simulink model "FDIteamUAV"  (R2018a)
settings: Solver=FixedStepAuto  StartTime=0.0  StopTime=100  FixedStep=0.1  RelTol=1e-3
InitFcn:
  | clear
  | close all
  | parameterVehicleControl
  | fdi_mask_init
values from neighbouring files (symbols this model uses):
  a = x_waypoint(1)+10    [parameterVehicleControl.m]
  a2 = x_waypoint(1)    [parameterVehicleControl.m]
  a3 = x_waypoint(1)-10    [parameterVehicleControl.m]
  b = y_waypoint(1)    [parameterVehicleControl.m]
  b2 = y_waypoint(1)    [parameterVehicleControl.m]
  b3 = y_waypoint(1)    [parameterVehicleControl.m]
  fdi_alarm_thrsld = 9.2103    [fdi_mask_init.m]
  fdi_duration_1_airs = 55    [fdi_mask_init.m]
  fdi_duration_2_airs = 1000    [fdi_mask_init.m]
  fdi_duration_3_airs = 0    [fdi_mask_init.m]
  fdi_fixed_matix_1_airs = fdi_fault_value_1_airs    (= 3)    [fdi_mask_init.m]
  fdi_fixed_matix_2_airs = fdi_fault_value_2_airs    (= 3)    [fdi_mask_init.m]
  fdi_fixed_matix_3_airs = fdi_fault_value_3_airs    (= 0)    [fdi_mask_init.m]
  fdi_gain_matrix_1_airs = 1    [fdi_mask_init.m]
  fdi_gain_matrix_2_airs = 1    [fdi_mask_init.m]
  fdi_gain_matrix_3_airs = 1    [fdi_mask_init.m]
  fdi_muNmu_1_airs = fdi_mu_1_airs/norm(fdi_mu_1_airs)    [fdi_mask_init.m]
  fdi_muNmu_2_airs = fdi_mu_2_airs/norm(fdi_mu_2_airs)    [fdi_mask_init.m]
  fdi_muNmu_3_airs = fdi_mu_3_airs/norm(fdi_mu_3_airs)    [fdi_mask_init.m]
  fdi_noise_var_airs = Noise_airs    (= 0.2)    [fdi_mask_init.m]
  fdi_seed_airs = ceil(rand(1,fdi_number_of_sensors)*1000)    [fdi_mask_init.m]
  fdi_SmT_airs = (fdi_V * fdi_R_airs * fdi_V')^(-1/2)    [fdi_mask_init.m]
  fdi_start_time_1_airs = 45    [fdi_mask_init.m]
  fdi_start_time_2_airs = 500    [fdi_mask_init.m]
  fdi_start_time_3_airs = 0    [fdi_mask_init.m]
  fdi_V = (null([1 1 1]))'    [fdi_mask_init.m]
  rl = 1*rNominal    (= 0.052959)    [parameterVehicleControl.m]
  rr = 1*rNominal    (= 0.052959)    [parameterVehicleControl.m]
  Tau2 = 1    [parameterVehicleControl.m]
  thetaIC = 90*(pi/180)    (= 1.57079632679)    [parameterVehicleControl.m]
  thetaIC2 = 90*(pi/180)    (= 1.57079632679)    [parameterVehicleControl.m]
  thetaIC3 = 90*(pi/180)    (= 1.57079632679)    [parameterVehicleControl.m]
  Ts = Tsample    [fdi_mask_init.m]
  Tsample = 1/10    (= 0.1)    [parameterVehicleControl.m]
  Vmax = 5    [parameterVehicleControl.m]
  xIC = 150    [parameterVehicleControl.m]
  xIC2 = 25    [parameterVehicleControl.m]
  xIC3 = -100    [parameterVehicleControl.m]
  yIC = 0    [parameterVehicleControl.m]
  yIC2 = 0    [parameterVehicleControl.m]
  yIC3 = 0    [parameterVehicleControl.m]
libraries: simulink x6
settings Model: Creator=hsevil  LastModifiedBy=hsevil
settings SolverCC: AlgebraicLoopSolver=LineSearch

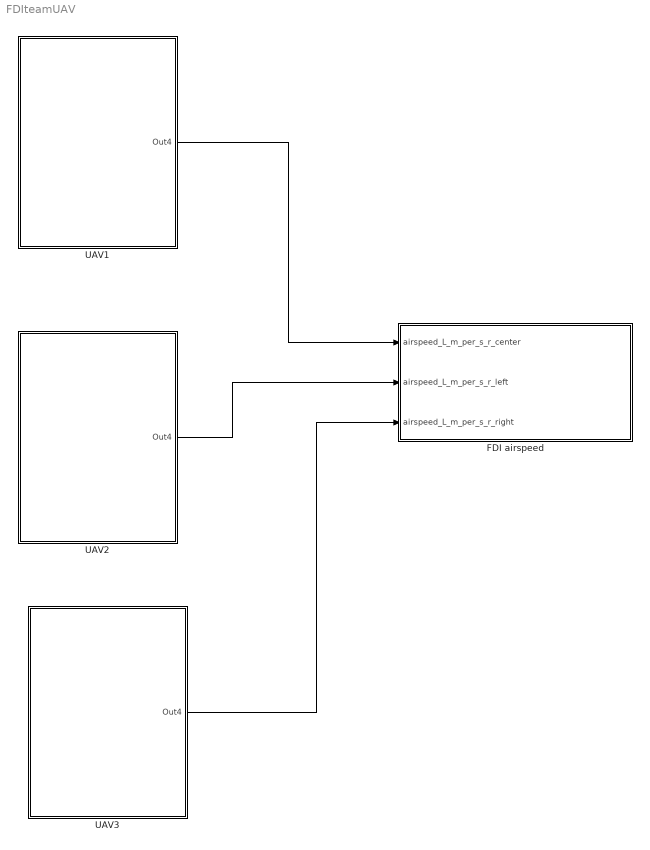
== system FDIteamUAV ==
  FDI airspeed : Subsystem
  UAV1 : Subsystem
  UAV2 : Subsystem
  UAV3 : Subsystem
  wires:
  UAV1/1(Out4) -> FDI airspeed/1(airspeed_L_m_per_s_r_center)
  UAV2/1(Out4) -> FDI airspeed/2(airspeed_L_m_per_s_r_left)
  UAV3/1(Out4) -> FDI airspeed/3(airspeed_L_m_per_s_r_right)

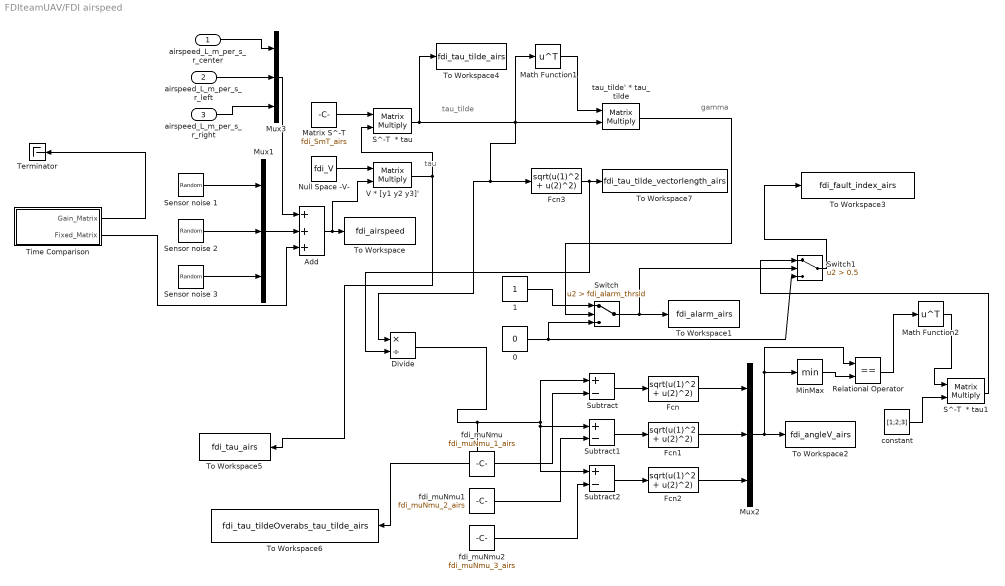
== system FDIteamUAV/FDI airspeed ==
  note: tau
  note: gamma
  note: tau_tilde
  airspeed_L_m_per_s_r_center : Inport
  airspeed_L_m_per_s_r_left : Inport  Port=2
  airspeed_L_m_per_s_r_right : Inport  Port=3
  0 : Constant  Value=0
  1 : Constant
  Add : Sum  Inputs=+++
  Divide : Product  Inputs=*/
  Fcn{,1..3} (4 alike) : Fcn  Expr=sqrt(u(1)^2 + u(2)^2)
  Math Function1 : Math  Operator=transpose  SaturateOnIntegerOverflow=on
  Math Function2 : Math  Operator=transpose  SaturateOnIntegerOverflow=on
  Matrix S^-T : Constant  Value=fdi_SmT_airs
  MinMax : MinMax
  Mux1 : Mux  Inputs=3
  Mux2 : Mux  Inputs=3
  Mux3 : Mux  Inputs=3
  Null Space -V- : Constant  Value=fdi_V
  Relational Operator : RelationalOperator  Operator===  OutDataTypeStr=boolean  RndMeth=Nearest
  S^-T  * tau : Product  Multiplication=Matrix(*)  RndMeth=Zero
  S^-T  * tau1 : Product  Multiplication=Matrix(*)  RndMeth=Zero
  Sensor noise 1 : RandomNumber  DisableCoverage=on  Variance=fdi_noise_var_airs  Seed=fdi_seed_airs(1)  SampleTime=Ts
  Sensor noise 2 : RandomNumber  DisableCoverage=on  Variance=fdi_noise_var_airs  Seed=fdi_seed_airs(2)  SampleTime=Ts
  Sensor noise 3 : RandomNumber  DisableCoverage=on  Variance=fdi_noise_var_airs  Seed=fdi_seed_airs(3)  SampleTime=Ts
  Subtract : Sum  Inputs=+-
  Subtract1 : Sum  Inputs=+-
  Subtract2 : Sum  Inputs=+-
  Switch : Switch  Criteria=u2 > Threshold  Threshold=fdi_alarm_thrsld
  Switch1 : Switch  Criteria=u2 > Threshold  Threshold=0.5
  Terminator : Terminator
  Time Comparison : Subsystem
  To Workspace : ToWorkspace  VariableName=fdi_airspeed  SampleTime=-1
  To Workspace1 : ToWorkspace  VariableName=fdi_alarm_airs  SampleTime=-1
  To Workspace2 : ToWorkspace  VariableName=fdi_angleV_airs  SampleTime=-1
  To Workspace3 : ToWorkspace  VariableName=fdi_fault_index_airs  SampleTime=-1
  To Workspace4 : ToWorkspace  VariableName=fdi_tau_tilde_airs  SampleTime=-1
  To Workspace5 : ToWorkspace  VariableName=fdi_tau_airs  SampleTime=-1
  To Workspace6 : ToWorkspace  VariableName=fdi_tau_tildeOverabs_tau_tilde_airs  SampleTime=-1
  To Workspace7 : ToWorkspace  VariableName=fdi_tau_tilde_vectorlength_airs  SampleTime=-1
  V * [y1 y2 y3]' : Product  Multiplication=Matrix(*)  RndMeth=Zero
  constant : Constant  Value=[1;2;3]
  fdi_muNmu : Constant  Value=fdi_muNmu_1_airs
  fdi_muNmu1 : Constant  Value=fdi_muNmu_2_airs
  fdi_muNmu2 : Constant  Value=fdi_muNmu_3_airs
  tau_tilde' * tau_tilde : Product  Multiplication=Matrix(*)  RndMeth=Zero
  wires:
  Sensor noise 1/1 -> Mux1/1
  Sensor noise 2/1 -> Mux1/2
  Sensor noise 3/1 -> Mux1/3
  Mux1/1 -> Add/2
  Mux3/1 -> Add/1
  Add/1 -> To Workspace/1, V * [y1 y2 y3]'/2
  Null Space -V-/1 -> V * [y1 y2 y3]'/1
  V * [y1 y2 y3]'/1 -> S^-T  * tau/2, To Workspace5/1
  Switch/1 -> To Workspace1/1, Switch1/2
  Math Function1/1 -> tau_tilde' * tau_tilde/1
  tau_tilde' * tau_tilde/1 -> Switch/2
  1/1 -> Switch/1
  0/1 -> Switch/3, Switch1/3
  S^-T  * tau/1 -> To Workspace4/1, Fcn3/1, Divide/1, tau_tilde' * tau_tilde/2, Math Function1/1
  Matrix S^-T/1 -> S^-T  * tau/1
  Subtract/1 -> Fcn/1
  Subtract1/1 -> Fcn1/1
  Subtract2/1 -> Fcn2/1
  Fcn/1 -> Mux2/1
  Fcn1/1 -> Mux2/2
  Fcn2/1 -> Mux2/3
  Mux2/1 -> To Workspace2/1, Relational Operator/1, MinMax/1
  fdi_muNmu/1 -> Subtract/2
  fdi_muNmu1/1 -> Subtract1/2
  fdi_muNmu2/1 -> Subtract2/2
  Switch1/1 -> To Workspace3/1
  MinMax/1 -> Relational Operator/2
  Relational Operator/1 -> Math Function2/1
  Math Function2/1 -> S^-T  * tau1/1
  constant/1 -> S^-T  * tau1/2
  S^-T  * tau1/1 -> Switch1/1
  airspeed_L_m_per_s_r_left/1 -> Mux3/2
  airspeed_L_m_per_s_r_right/1 -> Mux3/3
  airspeed_L_m_per_s_r_center/1 -> Mux3/1
  Fcn3/1 -> Divide/2, To Workspace7/1
  Divide/1 -> Subtract/1, Subtract1/1, Subtract2/1, To Workspace6/1
  Time Comparison/1(Gain_Matrix) -> Terminator/1
  Time Comparison/2(Fixed_Matrix) -> Add/3

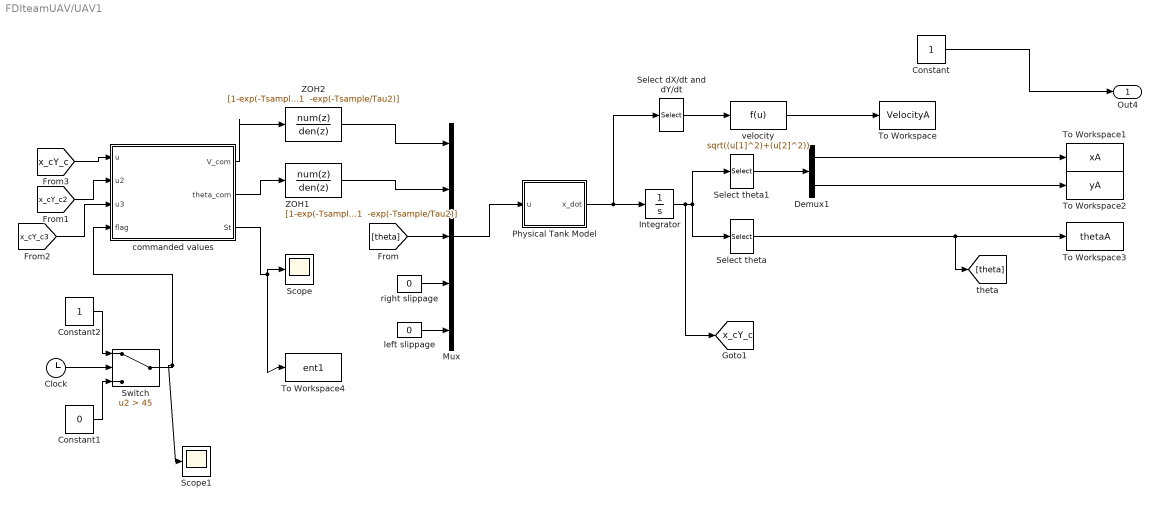
== system FDIteamUAV/UAV1 ==
  Clock : Clock
  Constant : Constant
  Constant1 : Constant  Value=0
  Constant2 : Constant
  Demux1 : Demux  Outputs=2
  Integrator : Integrator  InitialCondition=[xIC; yIC; thetaIC]
  Mux : Mux  Inputs=5
  Physical Tank Model : MATLAB Function  TreatAsAtomicUnit=on
  Scope : Scope
  Scope1 : Scope
  Select dX/dt and dY/dt : Selector  InputPortWidth=3  IndexOptions=Index vector (dialog)  Indices=[1 2]  OutputSizes=1
  Select theta : Selector  InputPortWidth=3  IndexOptions=Index vector (dialog)  Indices=3  OutputSizes=1
  Select theta1 : Selector  InputPortWidth=3  IndexOptions=Index vector (dialog)  Indices=[1 2]  OutputSizes=1
  Switch : Switch  Criteria=u2 > Threshold  Threshold=45
  To Workspace : ToWorkspace  VariableName=VelocityA  SampleTime=-1
      settings: Save2DSignal=2-D array (concatenate along first dimension)
  To Workspace1 : ToWorkspace  VariableName=xA  SampleTime=-1
      settings: Save2DSignal=2-D array (concatenate along first dimension)
  To Workspace2 : ToWorkspace  VariableName=yA  SampleTime=-1
      settings: Save2DSignal=2-D array (concatenate along first dimension)
  To Workspace3 : ToWorkspace  VariableName=thetaA  SampleTime=-1
      settings: Save2DSignal=2-D array (concatenate along first dimension)
  To Workspace4 : ToWorkspace  VariableName=ent1  SampleTime=-1
      settings: Save2DSignal=2-D array (concatenate along first dimension)
  ZOH1 : DiscreteTransferFcn  Numerator=[1-exp(-Tsample/Tau2)]  Denominator="[1  -exp(-Tsample/Tau2)]"  SampleTime=Tsample
  ZOH2 : DiscreteTransferFcn  Numerator=[1-exp(-Tsample/Tau2)]  Denominator="[1  -exp(-Tsample/Tau2)]"  SampleTime=Tsample
  commanded values : MATLAB Function  TreatAsAtomicUnit=on
  left slippage : Constant  Value=0
  "right slippage " : Constant  Value=0
  velocity : Fcn  Expr=sqrt((u[1]^2)+(u[2]^2))
  Out4 : Outport
  tag scope: x_cY_c=global
  wires:
  [x_cY_c] -> commanded values/1(u)
  Integrator/1 -> [x_cY_c], Select theta/1, Select theta1/1
  [theta] -> Mux/3
  commanded values/1(V_com) -> ZOH2/1
  commanded values/2(theta_com) -> ZOH1/1
  Demux1/1 -> To Workspace1/1
  Demux1/2 -> To Workspace2/1
  velocity/1 -> To Workspace/1
  Select theta/1 -> To Workspace3/1, [theta]
  Physical Tank Model/1(x_dot) -> Integrator/1, Select dX/dt and dY/dt/1
  "right slippage "/1 -> Mux/4
  ZOH1/1 -> Mux/2
  Select theta1/1 -> Demux1/1
  Select dX/dt and dY/dt/1 -> velocity/1
  left slippage/1 -> Mux/5
  Mux/1 -> Physical Tank Model/1(u)
  [x_cY_c2] -> commanded values/2(u2)
  [x_cY_c3] -> commanded values/3(u3)
  commanded values/3(St) -> To Workspace4/1, Scope/1
  ZOH2/1 -> Mux/1
  Constant/1 -> Out4/1
  Clock/1 -> Switch/2
  Constant1/1 -> Switch/3
  Constant2/1 -> Switch/1
  Switch/1 -> Scope1/1, commanded values/4(flag)

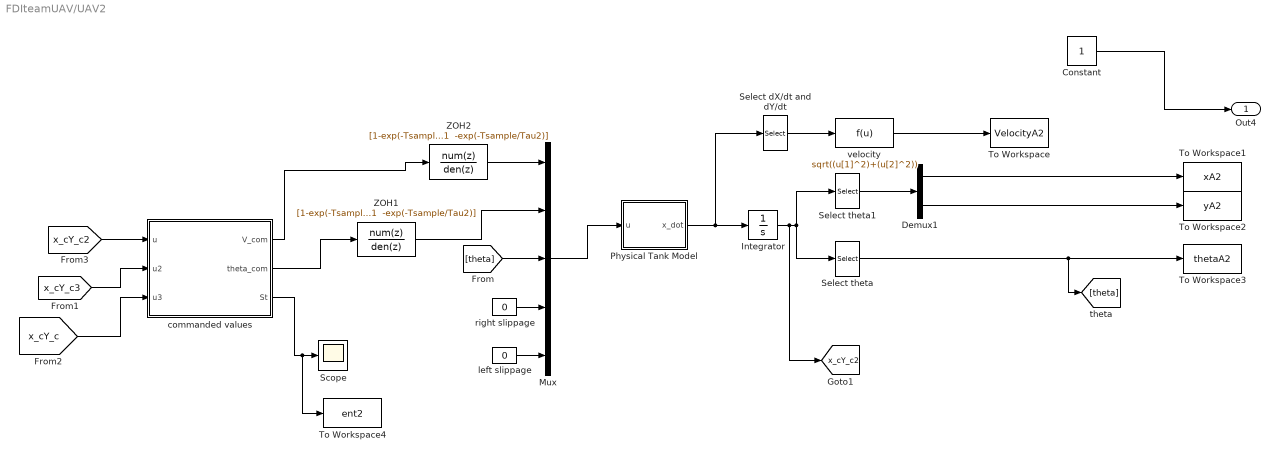
== system FDIteamUAV/UAV2 ==
  Constant : Constant
  Demux1 : Demux  Outputs=2
  Integrator : Integrator  InitialCondition=[xIC2; yIC2 ; thetaIC2]
  Mux : Mux  Inputs=5
  Physical Tank Model : MATLAB Function  TreatAsAtomicUnit=on
  Scope : Scope
  Select dX/dt and dY/dt : Selector  InputPortWidth=3  IndexOptions=Index vector (dialog)  Indices=[1 2]  OutputSizes=1
  Select theta : Selector  InputPortWidth=3  IndexOptions=Index vector (dialog)  Indices=3  OutputSizes=1
  Select theta1 : Selector  InputPortWidth=3  IndexOptions=Index vector (dialog)  Indices=[1 2]  OutputSizes=1
  To Workspace : ToWorkspace  VariableName=VelocityA2  SampleTime=-1
      settings: Save2DSignal=2-D array (concatenate along first dimension)
  To Workspace1 : ToWorkspace  VariableName=xA2  SampleTime=-1
      settings: Save2DSignal=2-D array (concatenate along first dimension)
  To Workspace2 : ToWorkspace  VariableName=yA2  SampleTime=-1
      settings: Save2DSignal=2-D array (concatenate along first dimension)
  To Workspace3 : ToWorkspace  VariableName=thetaA2  SampleTime=-1
      settings: Save2DSignal=2-D array (concatenate along first dimension)
  To Workspace4 : ToWorkspace  VariableName=ent2  SampleTime=-1
      settings: Save2DSignal=2-D array (concatenate along first dimension)
  ZOH1 : DiscreteTransferFcn  Numerator=[1-exp(-Tsample/Tau2)]  Denominator="[1  -exp(-Tsample/Tau2)]"  SampleTime=Tsample
  ZOH2 : DiscreteTransferFcn  Numerator=[1-exp(-Tsample/Tau2)]  Denominator="[1  -exp(-Tsample/Tau2)]"  SampleTime=Tsample
  commanded values : MATLAB Function  TreatAsAtomicUnit=on
  left slippage : Constant  Value=0
  "right slippage " : Constant  Value=0
  velocity : Fcn  Expr=sqrt((u[1]^2)+(u[2]^2))
  Out4 : Outport
  tag scope: x_cY_c2=global
  wires:
  [x_cY_c2] -> commanded values/1(u)
  Integrator/1 -> [x_cY_c2], Select theta/1, Select theta1/1
  [theta] -> Mux/3
  commanded values/1(V_com) -> ZOH2/1
  commanded values/2(theta_com) -> ZOH1/1
  Demux1/1 -> To Workspace1/1
  Demux1/2 -> To Workspace2/1
  velocity/1 -> To Workspace/1
  Select theta/1 -> To Workspace3/1, [theta]
  Physical Tank Model/1(x_dot) -> Integrator/1, Select dX/dt and dY/dt/1
  "right slippage "/1 -> Mux/4
  ZOH1/1 -> Mux/2
  Select theta1/1 -> Demux1/1
  Select dX/dt and dY/dt/1 -> velocity/1
  left slippage/1 -> Mux/5
  Mux/1 -> Physical Tank Model/1(u)
  [x_cY_c3] -> commanded values/2(u2)
  [x_cY_c] -> commanded values/3(u3)
  commanded values/3(St) -> To Workspace4/1, Scope/1
  ZOH2/1 -> Mux/1
  Constant/1 -> Out4/1

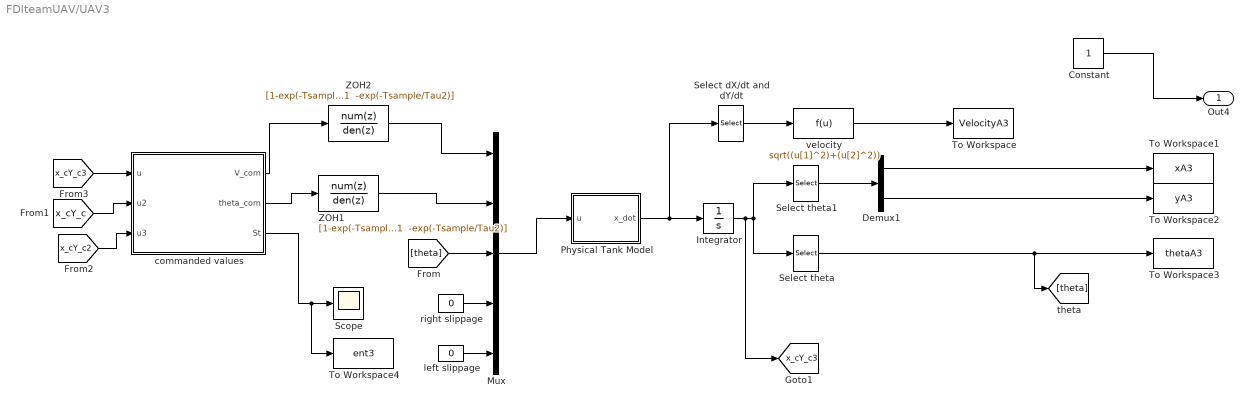
== system FDIteamUAV/UAV3 ==
  Constant : Constant
  Demux1 : Demux  Outputs=2
  Integrator : Integrator  InitialCondition=[xIC3; yIC3; thetaIC3]
  Mux : Mux  Inputs=5
  Physical Tank Model : MATLAB Function  TreatAsAtomicUnit=on
  Scope : Scope
  Select dX/dt and dY/dt : Selector  InputPortWidth=3  IndexOptions=Index vector (dialog)  Indices=[1 2]  OutputSizes=1
  Select theta : Selector  InputPortWidth=3  IndexOptions=Index vector (dialog)  Indices=3  OutputSizes=1
  Select theta1 : Selector  InputPortWidth=3  IndexOptions=Index vector (dialog)  Indices=[1 2]  OutputSizes=1
  To Workspace : ToWorkspace  VariableName=VelocityA3  SampleTime=-1
      settings: Save2DSignal=2-D array (concatenate along first dimension)
  To Workspace1 : ToWorkspace  VariableName=xA3  SampleTime=-1
      settings: Save2DSignal=2-D array (concatenate along first dimension)
  To Workspace2 : ToWorkspace  VariableName=yA3  SampleTime=-1
      settings: Save2DSignal=2-D array (concatenate along first dimension)
  To Workspace3 : ToWorkspace  VariableName=thetaA3  SampleTime=-1
      settings: Save2DSignal=2-D array (concatenate along first dimension)
  To Workspace4 : ToWorkspace  VariableName=ent3  SampleTime=-1
      settings: Save2DSignal=2-D array (concatenate along first dimension)
  ZOH1 : DiscreteTransferFcn  Numerator=[1-exp(-Tsample/Tau2)]  Denominator="[1  -exp(-Tsample/Tau2)]"  SampleTime=Tsample
  ZOH2 : DiscreteTransferFcn  Numerator=[1-exp(-Tsample/Tau2)]  Denominator="[1  -exp(-Tsample/Tau2)]"  SampleTime=Tsample
  commanded values : MATLAB Function  TreatAsAtomicUnit=on
  left slippage : Constant  Value=0
  "right slippage " : Constant  Value=0
  velocity : Fcn  Expr=sqrt((u[1]^2)+(u[2]^2))
  Out4 : Outport
  tag scope: x_cY_c3=global
  wires:
  [x_cY_c3] -> commanded values/1(u)
  Integrator/1 -> [x_cY_c3], Select theta/1, Select theta1/1
  [theta] -> Mux/3
  commanded values/1(V_com) -> ZOH2/1
  commanded values/2(theta_com) -> ZOH1/1
  Demux1/1 -> To Workspace1/1
  Demux1/2 -> To Workspace2/1
  velocity/1 -> To Workspace/1
  Select theta/1 -> To Workspace3/1, [theta]
  Physical Tank Model/1(x_dot) -> Integrator/1, Select dX/dt and dY/dt/1
  "right slippage "/1 -> Mux/4
  ZOH1/1 -> Mux/2
  Select theta1/1 -> Demux1/1
  Select dX/dt and dY/dt/1 -> velocity/1
  left slippage/1 -> Mux/5
  Mux/1 -> Physical Tank Model/1(u)
  [x_cY_c] -> commanded values/2(u2)
  [x_cY_c2] -> commanded values/3(u3)
  commanded values/3(St) -> To Workspace4/1, Scope/1
  ZOH2/1 -> Mux/1
  Constant/1 -> Out4/1

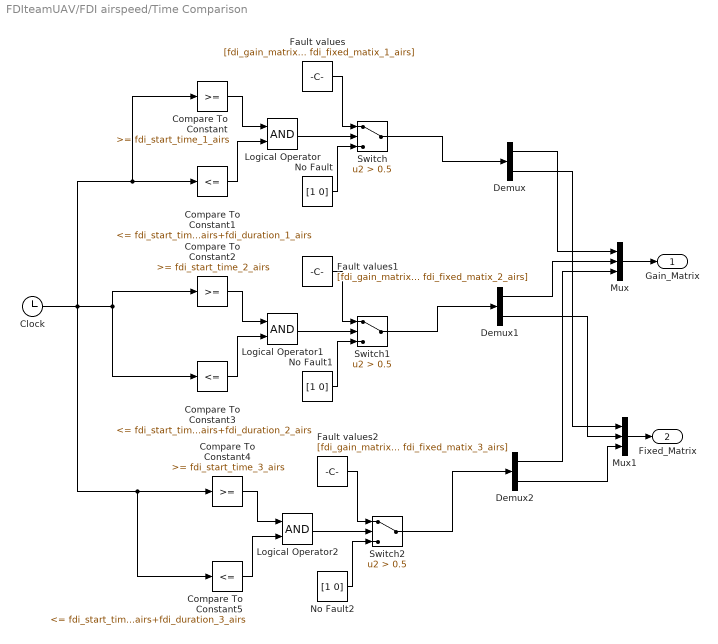
== system FDIteamUAV/FDI airspeed/Time Comparison ==
  Clock : Clock
  Compare To Constant : simulink/Logic and Bit Operations/Compare To Constant  relop=>=  const=fdi_start_time_1_airs  OutDataTypeStr=uint8  ZeroCross=off
  Compare To Constant1 : simulink/Logic and Bit Operations/Compare To Constant  relop=<=  const=fdi_start_time_1_airs+fdi_duration_1_airs  OutDataTypeStr=uint8  ZeroCross=off
  Compare To Constant2 : simulink/Logic and Bit Operations/Compare To Constant  relop=>=  const=fdi_start_time_2_airs  OutDataTypeStr=uint8  ZeroCross=off
  Compare To Constant3 : simulink/Logic and Bit Operations/Compare To Constant  relop=<=  const=fdi_start_time_2_airs+fdi_duration_2_airs  OutDataTypeStr=uint8  ZeroCross=off
  Compare To Constant4 : simulink/Logic and Bit Operations/Compare To Constant  relop=>=  const=fdi_start_time_3_airs  OutDataTypeStr=uint8  ZeroCross=off
  Compare To Constant5 : simulink/Logic and Bit Operations/Compare To Constant  relop=<=  const=fdi_start_time_3_airs+fdi_duration_3_airs  OutDataTypeStr=uint8  ZeroCross=off
  Demux : Demux  Outputs=2
  Demux1 : Demux  Outputs=2
  Demux2 : Demux  Outputs=2
  Fault values : Constant  Value=[fdi_gain_matrix_1_airs fdi_fixed_matix_1_airs]
  Fault values1 : Constant  Value=[fdi_gain_matrix_2_airs fdi_fixed_matix_2_airs]
  Fault values2 : Constant  Value=[fdi_gain_matrix_3_airs fdi_fixed_matix_3_airs]
  Logical Operator : Logic  AllPortsSameDT=off  OutDataTypeStr=boolean
  Logical Operator1 : Logic  AllPortsSameDT=off  OutDataTypeStr=boolean
  Logical Operator2 : Logic  AllPortsSameDT=off  OutDataTypeStr=boolean
  Mux : Mux  Inputs=3
  Mux1 : Mux  Inputs=3
  No Fault : Constant  Value=[1 0]
  No Fault1 : Constant  Value=[1 0]
  No Fault2 : Constant  Value=[1 0]
  Switch : Switch  Criteria=u2 > Threshold  Threshold=0.5
  Switch1 : Switch  Criteria=u2 > Threshold  Threshold=0.5
  Switch2 : Switch  Criteria=u2 > Threshold  Threshold=0.5
  Gain_Matrix : Outport
  Fixed_Matrix : Outport  Port=2
  wires:
  Demux/1 -> Mux/1
  Demux1/1 -> Mux/2
  Demux2/1 -> Mux/3
  Demux/2 -> Mux1/1
  Demux1/2 -> Mux1/2
  Demux2/2 -> Mux1/3
  Compare To Constant1/1 -> Logical Operator/2
  Compare To Constant/1 -> Logical Operator/1
  Logical Operator/1 -> Switch/2
  No Fault/1 -> Switch/3
  Fault values/1 -> Switch/1
  Mux/1 -> Gain_Matrix/1
  Mux1/1 -> Fixed_Matrix/1
  Compare To Constant3/1 -> Logical Operator1/2
  Compare To Constant2/1 -> Logical Operator1/1
  Logical Operator1/1 -> Switch1/2
  No Fault1/1 -> Switch1/3
  Fault values1/1 -> Switch1/1
  Compare To Constant5/1 -> Logical Operator2/2
  Compare To Constant4/1 -> Logical Operator2/1
  Logical Operator2/1 -> Switch2/2
  No Fault2/1 -> Switch2/3
  Fault values2/1 -> Switch2/1
  Clock/1 -> Compare To Constant2/1, Compare To Constant3/1, Compare To Constant1/1, Compare To Constant/1, Compare To Constant4/1, Compare To Constant5/1
  Switch/1 -> Demux/1
  Switch1/1 -> Demux1/1
  Switch2/1 -> Demux2/1

== matlab function FDIteamUAV/UAV1/Physical Tank Model ==
  data: u input; x_dot output size=[3,1]; b parameter; rr parameter; rl parameter
function x_dot = fcn(u,b,rr,rl)
%#eml

wr = u(1);
wl = u(2);
theta = u(3);
sr = u(4);
sl = u(5);
% x_dot = [((1-sr)*rr*wr + (1-sl)*rl*wl)*cos(theta)/2;
%          ((1-sr)*rr*wr + (1-sl)*rl*wl)*sin(theta)/2;
%          ((1-sl)*rl*wl - (1-sr)*rr*wr)/b];

     x_dot = [wr*cos(theta);
         wr*sin(theta);
         wl];
     
end

== matlab function FDIteamUAV/UAV1/commanded values ==
  data: V_com output; u input; u2 input; u3 input; theta_com output; a parameter; b parameter; Vmax parameter; St output; flag input
function [V_com,theta_com,St] = fcn(u,u2,u3,a,b,Vmax,flag)
x=zeros(3);
y=zeros(3);
t=zeros(3);
d=zeros(3);
Th=zeros(3);
V_com=0;
theta_com=0;
e=zeros(3);

if flag==1
    a=a+190;
end

x_cur=u(1);
y_cur=u(2);
theta_cur=u(3);

x(2)=u2(1);
y(2)=u2(2);
t(2)=u2(3);

x(3)=u3(1);
y(3)=u3(2);
t(3)=u3(3);

d(2)=sqrt((x(2)-x_cur)^2+(y(2)-y_cur)^2);
Th(2)=atan2( (y(2)-y_cur), (x(2)-x_cur) );

d(3)=sqrt((x(3)-x_cur)^2+(y(3)-y_cur)^2);
Th(3)=atan2( (y(3)-y_cur), (x(3)-x_cur) );

if d(2)<d(3)
    min=d(2);
    max=d(3);
    index=2;
    index2=3;
else
    min=d(3);
    max=d(2);
    index=3;
    index2=2;
end

for i=2:3
    if (100-d(i))<0
        e(i)=0;
    elseif (100-d(i))>25
        e(i)=25;
    end
end
%entropy
Threshold=1;
q=0.5;
sum= ( (e(2)/100)^q ) + ( (e(3)/100)^q );
St=(1-sum)/(1-q);
St_temp=St;

xd=(a-x_cur); 
yd=(b-y_cur); 
 
d_left = sqrt(xd^2+yd^2);

theta_targ=atan2(yd,xd);

if flag==1
    St=0.5;
    min=11;
end

if St<Threshold
    
    if min>10
    
        theta_com=(theta_targ-theta_cur);
        if theta_com>pi
            theta_com=-2*pi+theta_com;
        elseif theta_com<-pi
            theta_com=2*pi+theta_com;
        end
        
        if d_left>100
            d_left=100;
        end
        
        V_com=Vmax;% * (d_left/100);
    
    else
        theta_com=(Th(index)-theta_cur) + pi;
        if theta_com>pi
            theta_com=-2*pi+theta_com + pi;
        elseif theta_com<-pi
            theta_com=2*pi+theta_com + pi;
            
        end
        
        if d(index)>100
            d(index)=100;
        end
        
        V_com=1/2 * Vmax;% * (d(index)/100);
    end
    
    
elseif min>10
        theta_com=(Th(index)-theta_cur);
    if theta_com>pi
        theta_com=-2*pi+theta_com;
    elseif theta_com<-pi
        theta_com=2*pi+theta_com;
    end
    
    if d(index)>100
        d(index)=100;
    end
    
    V_com=1/2 * Vmax;% * (d(index)/100);
    
elseif max>10
            theta_com=(Th(index2)-theta_cur);
    if theta_com>pi
        theta_com=-2*pi+theta_com;
    elseif theta_com<-pi
        theta_com=2*pi+theta_com;
    end
    
    if d(index2)>100
        d(index2)=100;
    end
    
    V_com=1/2 * Vmax;% * (d(index2)/100);
    
elseif min<10 || max<10
            theta_com=(Th(index)-theta_cur) + pi;
    if theta_com>pi
        theta_com=-2*pi+theta_com + pi;
    elseif theta_com<-pi
        theta_com=2*pi+theta_com + pi;

    end
    
    if d(index)>100
        d(index)=100;
    end
    
    V_com=2 * Vmax;% * (d(index)/100);
    
end

St=St_temp;

== matlab function FDIteamUAV/UAV2/Physical Tank Model ==
  data: u input; x_dot output size=[3,1]; b parameter; rr parameter; rl parameter
function x_dot = fcn(u,b,rr,rl)
%#eml

wr = u(1);
wl = u(2);
theta = u(3);
sr = u(4);
sl = u(5);
% x_dot = [((1-sr)*rr*wr + (1-sl)*rl*wl)*cos(theta)/2;
%          ((1-sr)*rr*wr + (1-sl)*rl*wl)*sin(theta)/2;
%          ((1-sl)*rl*wl - (1-sr)*rr*wr)/b];

     x_dot = [wr*cos(theta);
         wr*sin(theta);
         wl];
     
end

== matlab function FDIteamUAV/UAV2/commanded values ==
  data: V_com output; u input; u2 input; u3 input; theta_com output; a2 parameter; b2 parameter; Vmax parameter; St output
function [V_com,theta_com,St] = fcn(u,u2,u3,a2,b2,Vmax)
x=zeros(3);
y=zeros(3);
t=zeros(3);
d=zeros(3);
Th=zeros(3);
V_com=0;
theta_com=0;
e=zeros(3);

x_cur=u(1);
y_cur=u(2);
theta_cur=u(3);

x(2)=u2(1);
y(2)=u2(2);
t(2)=u2(3);

x(3)=u3(1);
y(3)=u3(2);
t(3)=u3(3);

d(2)=sqrt((x(2)-x_cur)^2+(y(2)-y_cur)^2);
Th(2)=atan2( (y(2)-y_cur), (x(2)-x_cur) );

d(3)=sqrt((x(3)-x_cur)^2+(y(3)-y_cur)^2);
Th(3)=atan2( (y(3)-y_cur), (x(3)-x_cur) );

if d(2)<d(3)
    min=d(2);
    max=d(3);
    index=2;
    index2=3;
else
    min=d(3);
    max=d(2);
    index=3;
    index2=2;
end

for i=2:3
    if (100-d(i))<0
        e(i)=0;
    elseif (100-d(i))>25
        e(i)=25;
    end
end
%entropy
Threshold=1;
q=0.5;
sum= ( (e(2)/100)^q ) + ( (e(3)/100)^q );
St=(1-sum)/(1-q);

xd=(a2-x_cur); 
yd=(b2-y_cur); 
 
d_left = sqrt(xd^2+yd^2);

theta_targ=atan2(yd,xd);

if St<Threshold
    
    if min>10
    
        theta_com=(theta_targ-theta_cur);
        if theta_com>pi
            theta_com=-2*pi+theta_com;
        elseif theta_com<-pi
            theta_com=2*pi+theta_com;
        end
        
        if d_left>100
            d_left=100;
        end
        
        V_com=Vmax;% * (d_left/100);
    
    else
        theta_com=(Th(index)-theta_cur) + pi;
        if theta_com>pi
            theta_com=-2*pi+theta_com + pi;
        elseif theta_com<-pi
            theta_com=2*pi+theta_com + pi;
            
        end
        
        if d(index)>100
            d(index)=100;
        end
        
        V_com=1/2 * Vmax;% * (d(index)/100);
    end
    
elseif min>10
        theta_com=(Th(index)-theta_cur);
    if theta_com>pi
        theta_com=-2*pi+theta_com;
    elseif theta_com<-pi
        theta_com=2*pi+theta_com;
    end
    
    if d(index)>100
        d(index)=100;
    end
    
    V_com=1/2 * Vmax;% * (d(index)/100);
    
elseif max>10
            theta_com=(Th(index2)-theta_cur);
    if theta_com>pi
        theta_com=-2*pi+theta_com;
    elseif theta_com<-pi
        theta_com=2*pi+theta_com;
    end
    
    if d(index2)>100
        d(index2)=100;
    end
    
    V_com=1/2 * Vmax;% * (d(index2)/100);
    
elseif min<10 || max<10
            theta_com=(Th(index)-theta_cur) + pi;
    if theta_com>pi
        theta_com=-2*pi+theta_com + pi;
    elseif theta_com<-pi
        theta_com=2*pi+theta_com + pi;

    end
    
    if d(index)>100
        d(index)=100;
    end
    
    V_com=2 * Vmax;% * (d(index)/100);
    
end

== matlab function FDIteamUAV/UAV3/Physical Tank Model ==
  data: u input; x_dot output size=[3,1]; b parameter; rr parameter; rl parameter
function x_dot = fcn(u,b,rr,rl)
%#eml

wr = u(1);
wl = u(2);
theta = u(3);
sr = u(4);
sl = u(5);
% x_dot = [((1-sr)*rr*wr + (1-sl)*rl*wl)*cos(theta)/2;
%          ((1-sr)*rr*wr + (1-sl)*rl*wl)*sin(theta)/2;
%          ((1-sl)*rl*wl - (1-sr)*rr*wr)/b];

     x_dot = [wr*cos(theta);
         wr*sin(theta);
         wl];
     
end

== matlab function FDIteamUAV/UAV3/commanded values ==
  data: V_com output; u input; u2 input; u3 input; theta_com output; a3 parameter; b3 parameter; Vmax parameter; St output
function [V_com,theta_com,St] = fcn(u,u2,u3,a3,b3,Vmax)
x=zeros(3);
y=zeros(3);
t=zeros(3);
d=zeros(3);
Th=zeros(3);
V_com=0;
theta_com=0;
e=zeros(3);

x_cur=u(1);
y_cur=u(2);
theta_cur=u(3);

x(2)=u2(1);
y(2)=u2(2);
t(2)=u2(3);

x(3)=u3(1);
y(3)=u3(2);
t(3)=u3(3);

d(2)=sqrt((x(2)-x_cur)^2+(y(2)-y_cur)^2);
Th(2)=atan2( (y(2)-y_cur), (x(2)-x_cur) );

d(3)=sqrt((x(3)-x_cur)^2+(y(3)-y_cur)^2);
Th(3)=atan2( (y(3)-y_cur), (x(3)-x_cur) );

if d(2)<d(3)
    min=d(2);
    max=d(3);
    index=2;
    index2=3;
else
    min=d(3);
    max=d(2);
    index=3;
    index2=2;
end

for i=2:3
    if (100-d(i))<0
        e(i)=0;
    elseif (100-d(i))>25
        e(i)=25;
    end
end
%entropy
Threshold=1;
q=0.5;
sum= ( (e(2)/100)^q ) + ( (e(3)/100)^q );
St=(1-sum)/(1-q);

xd=(a3-x_cur); 
yd=(b3-y_cur); 
 
d_left = sqrt(xd^2+yd^2);

theta_targ=atan2(yd,xd);

if St<Threshold
    
    if min>10
    
        theta_com=(theta_targ-theta_cur);
        if theta_com>pi
            theta_com=-2*pi+theta_com;
        elseif theta_com<-pi
            theta_com=2*pi+theta_com;
        end
        
        if d_left>100
            d_left=100;
        end
        
        V_com=Vmax;% * (d_left/100);
    
    else
        theta_com=(Th(index)-theta_cur) + pi;
        if theta_com>pi
            theta_com=-2*pi+theta_com + pi;
        elseif theta_com<-pi
            theta_com=2*pi+theta_com + pi;
            
        end
        
        if d(index)>100
            d(index)=100;
        end
        
        V_com=1 * Vmax;% * (d(index)/100);
    end
    
elseif min>10
        theta_com=(Th(index)-theta_cur);
    if theta_com>pi
        theta_com=-2*pi+theta_com;
    elseif theta_com<-pi
        theta_com=2*pi+theta_com;
    end
    
    if d(index)>100
        d(index)=100;
    end
    
    V_com=1 * Vmax;% * (d(index)/100);
    
elseif max>10
            theta_com=(Th(index2)-theta_cur);
    if theta_com>pi
        theta_com=-2*pi+theta_com;
    elseif theta_com<-pi
        theta_com=2*pi+theta_com;
    end
    
    if d(index2)>100
        d(index2)=100;
    end
    
    V_com=1 * Vmax;% * (d(index2)/100);
    
elseif min<10 || max<10
            theta_com=(Th(index)-theta_cur) + pi;
    if theta_com>pi
        theta_com=-2*pi+theta_com + pi;
    elseif theta_com<-pi
        theta_com=2*pi+theta_com + pi;

    end
    
    if d(index)>100
        d(index)=100;
    end
    
    V_com=2 * Vmax;% * (d(index)/100);
    
end
